simulink model "EENG650assignment2"  (R2020b)
settings: Solver=VariableStepAuto  StartTime=0.0  StopTime=10.0  RelTol=1e-3
settings Model: EnablePacing=on  PacingRate=0.450000  Creator=Kelvin  LastModifiedBy=Kelvin

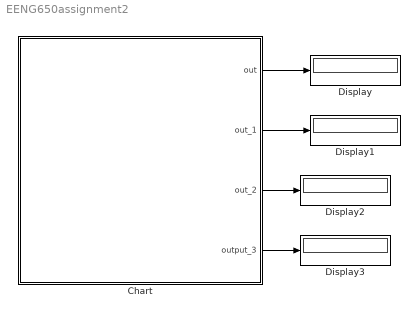
== system EENG650assignment2 ==
  Chart : Stateflow chart  TreatAsAtomicUnit=on
  Display{,1..3} (4 alike) : Display
  wires:
  Chart/1(out) -> Display/1
  Chart/2(out_1) -> Display1/1
  Chart/3(out_2) -> Display2/1
  Chart/4(output_3) -> Display3/1

== stateflow chart EENG650assignment2/Chart ==
  note: Note set run speed to .45sec to see every itteration
      |
      | First, it loops through state 1 -> state2 -> state 8
      | for 4 increments.
      |
      |  it goes to state 4 then to state 5
      | where it stays for 2 increments then it
      | precedes to state 6 where it stays for 8
      | increments
      | afterward, it stays in state 7 for  2
      | increments
      | finally, it ends at the junction END.
  state State1
  state Sate7
  state State0
  state State2
    entry:
    out = X;
  note: return hand-set
  note: END
  note: Dead
  note: Talk
  note: Start
  note: Wait
  state State3
  state State4
    entry:
    out_1 = y;
  state State5
    entry:
    out_2 = x;
  state State6
    entry:
    output_3 = Y;
  note: Play text
  note: Beep
  note: Record
  note: Beep
  Sate7 -> State1 [order 1] : {X = X+1;}
  (default) -> State0
  State2 -> Sate7
  Sate7 -> (junction 55) [order 2]
  State0 -> (junction 4)
  (junction 4) -> State1 : {X =0;}
  State1 -> State2 [order 1] : [X<=5]
  State6 -> (junction 55) [order 2] : [Y>=1]
  State1 -> State3 [order 2] : [X>=4]
  State6 -> (junction 46) [order 1] : {Y = Y+1;}
  (junction 19) -> State4 : [y<=2]
  State4 -> (junction 41) [order 1] : [y>=1]
      | {x=0;}
  (junction 41) -> State5 : [x<=9]
  State5 -> (junction 46) [order 2] : [x>=8]
      | {Y=0;}
  (junction 46) -> State6 : [Y<=2]
  State3 -> (junction 19) : {y=0;}
  State5 -> (junction 41) [order 1] : {x = x+1;}
  State4 -> (junction 19) [order 2] : {y = y+1;}
  data: X local; out output; y local; out_1 output; x local; out_2 output; Y local; output_3 output
